simulink model "ereg_single_tank"  (R2025a)
settings: Solver=VariableStepAuto  StartTime=0.0  StopTime=10  FixedStep=0.00001  MaxStep=0.002  RelTol=1e-3
values from neighbouring files (symbols this model uses):
  A_1_4_tube = id_2_A(id_1_4_tube)    [ereg_sim.m]    (also in ereg_system_sim_run.m)
  A_fuel_ullage_port = A_1_4_tube    [ereg_sim.m]    (also in ereg_system_sim_run.m)
  A_ox_ullage_port = A_1_4_tube    [ereg_sim.m]    (also in ereg_system_sim_run.m)
  fuel_init_P = 50e5    (= 5000000)    [ereg_sim.m]    (also in ereg_system_sim_run.m)
  ox_feed_CdA = 45e-6    (= 4.5e-05)    [ereg_sim.m]    (also in ereg_system_sim_run.m)
  ox_init_P = 50e5    (= 5000000)    [ereg_sim.m]    (also in ereg_system_sim_run.m)
  rho_fuel = 790    [ereg_sim.m]    (also in ereg_system_sim_run.m)
  rho_ox = 950    [ereg_sim.m]    (also in ereg_system_sim_run.m)
libraries: nesl_utility x33, fl_lib x32, SimscapeFluids_lib x8
(part 2 of 2)

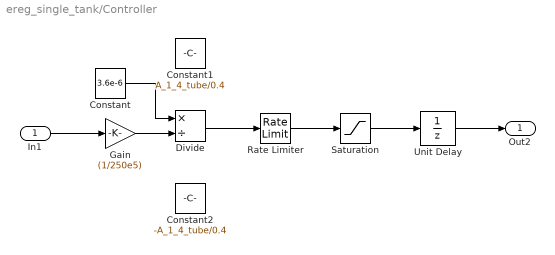
== system ereg_single_tank/Controller ==
  In1 : Inport
  Constant : Constant  Value=3.6e-6
  Constant1 : Constant  Value=A_1_4_tube/0.4
  Constant2 : Constant  Value=-A_1_4_tube/0.4
  Divide : Product  Inputs=*/
  Gain : Gain  Gain=(1/250e5)
  Rate Limiter : RateLimiter  RisingSlewLimit=A_1_4_tube/0.4  FallingSlewLimit=-A_1_4_tube/0.4  SampleTimeMode=inherited
  Saturation : Saturate  UpperLimit=A_1_4_tube  LowerLimit=0
  Unit Delay : UnitDelay  InitialCondition=3.6e-6  SampleTime=-1  HasFrameUpgradeWarning=on
  Out2 : Outport
  wires:
  In1/1 -> Gain/1
  Gain/1 -> Divide/2
  Constant/1 -> Divide/1
  Rate Limiter/1 -> Saturation/1
  Divide/1 -> Rate Limiter/1
  Unit Delay/1 -> Out2/1
  Saturation/1 -> Unit Delay/1

== matlab function ereg_single_tank/MATLAB Function1 ==
  data: mdot input; pc output
function pc = fcn(mdot)
    mdot = -mdot;
    if mdot > 0
        pc = ((mdot/2.33) * (30.8e5)) + 101325;
    else
        pc = 101325;
    end

== matlab function ereg_single_tank/MATLAB Function ==
  data: p_tank input; pc output; p_inj input; feed_CdA input; rho input
function pc = fcn(p_tank, p_inj, feed_CdA, rho)
    if p_tank > p_inj
        mdot = feed_CdA * sqrt(2 * rho * (p_tank - p_inj));
        pc = ((mdot/2.33) * (30.8e5)) + 101325;
    else
        pc = 101325;
    end
    pc = pc;
